simulink model "Kinematic_Delta_Robot"  (R2018b)
settings: Solver=VariableStepAuto  StartTime=0.0  StopTime=2  RelTol=1e-3
settings Model: Creator=User  LastModifiedBy=hugol
settings DebuggingCC: LibraryContextMissingDiagnostic=none
settings SFSimCC: SimUseLocalCustomCode=off
settings RTWCC: RTWUseLocalCustomCode=off
settings CodeAppCC: StateflowObjectComments=on

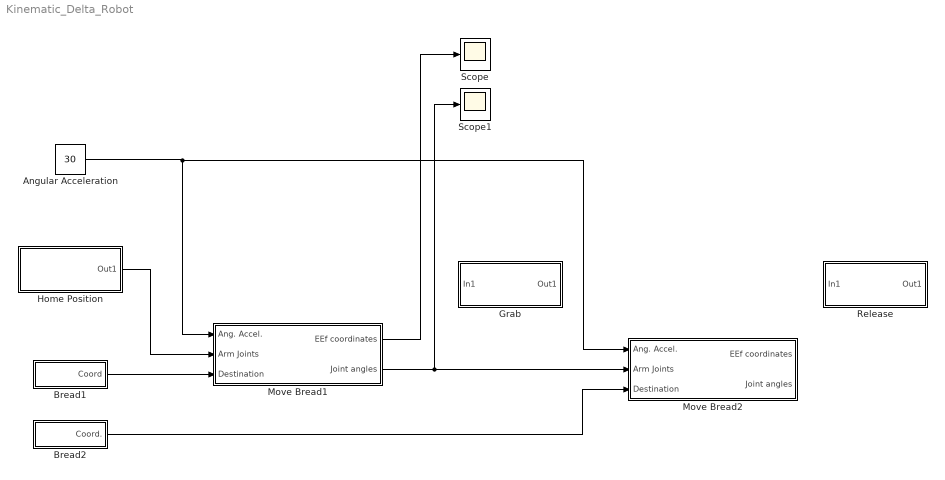
== system Kinematic_Delta_Robot ==
  Angular Acceleration : Constant  Value=30
  Bread1 : Subsystem
  Bread2 : Subsystem
  Grab : Subsystem
  Home Position : Subsystem
  Move Bread1 : Subsystem
  Move Bread2 : Subsystem
  Release : Subsystem
  Scope : Scope
  Scope1 : Scope
  wires:
  Bread1/1(Coord) -> Move Bread1/3(Destination)
  Home Position/1(Out1) -> Move Bread1/2(Arm Joints)
  Angular Acceleration/1 -> Move Bread2/1(Ang. Accel.), Move Bread1/1(Ang. Accel.)
  Bread2/1(Coord.) -> Move Bread2/3(Destination)
  Move Bread1/2(Joint angles) -> Scope1/1, Move Bread2/2(Arm Joints)
  Move Bread1/1(EEf coordinates) -> Scope/1

== system Kinematic_Delta_Robot/Bread1 ==
  Bread1.x : Constant  Value=48
  Bread1.y : Constant  Value=-25
  Bread1.z : Constant  Value=-400
  Mux : Mux  Inputs=3
  Coord : Outport
  wires:
  Bread1.y/1 -> Mux/2
  Bread1.z/1 -> Mux/3
  Bread1.x/1 -> Mux/1
  Mux/1 -> Coord/1

== system Kinematic_Delta_Robot/Bread2 ==
  Bread1.x : Constant  Value=48
  Bread1.y : Constant  Value=25
  Bread1.z : Constant  Value=-400
  Mux : Mux  Inputs=3
  Coord. : Outport
  wires:
  Bread1.y/1 -> Mux/2
  Bread1.z/1 -> Mux/3
  Bread1.x/1 -> Mux/1
  Mux/1 -> Coord./1

== system Kinematic_Delta_Robot/Grab ==
  In1 : Inport
  Out1 : Outport
  wires:
  In1/1 -> Out1/1

== system Kinematic_Delta_Robot/Home Position ==
  Arm1 : Constant  Value=0
  Arm2 : Constant  Value=-10
  Arm3 : Constant  Value=-5
  Mux : Mux  Inputs=3
  Out1 : Outport
  wires:
  Arm1/1 -> Mux/1
  Arm2/1 -> Mux/2
  Arm3/1 -> Mux/3
  Mux/1 -> Out1/1

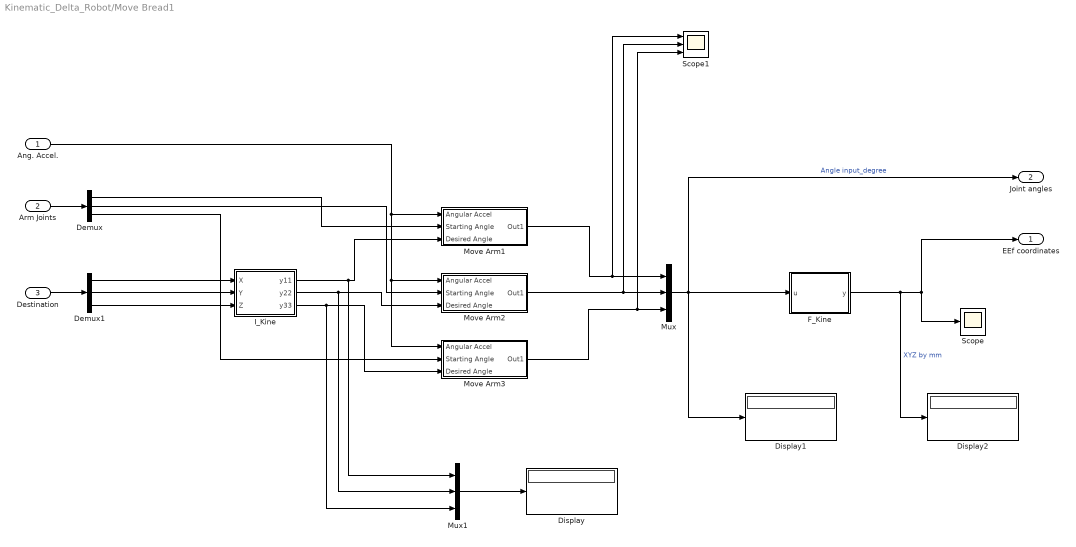
== system Kinematic_Delta_Robot/Move Bread1 ==
  Ang. Accel. : Inport
  Arm Joints : Inport  Port=2
  Destination : Inport  Port=3
  Demux : Demux  Outputs=3
  Demux1 : Demux  Outputs=3
  Display : Display
  Display1 : Display
  Display2 : Display
  F_Kine : MATLAB Function  TreatAsAtomicUnit=on
  I_Kine : MATLAB Function  TreatAsAtomicUnit=on
  Move Arm1 : Subsystem
  Move Arm2 : Subsystem
  Move Arm3 : Subsystem
  Mux : Mux  Inputs=3
  Mux1 : Mux  Inputs=3
  Scope : Scope
  Scope1 : Scope  NumInputPorts=3
  EEf coordinates : Outport
  Joint angles : Outport  Port=2
  wires:
  I_Kine/1(y11) -> Mux1/1, Move Arm1/3(Desired Angle)
  Demux/1 -> Move Arm1/2(Starting Angle)
  Move Arm3/1(Out1) -> Scope1/3, Mux/3
  Demux/2 -> Move Arm2/2(Starting Angle)
  Ang. Accel./1 -> Move Arm2/1(Angular Accel), Move Arm3/1(Angular Accel), Move Arm1/1(Angular Accel)
  Move Arm2/1(Out1) -> Scope1/2, Mux/2
  Move Arm1/1(Out1) -> Scope1/1, Mux/1
  Demux/3 -> Move Arm3/2(Starting Angle)
  I_Kine/2(y22) -> Move Arm2/3(Desired Angle), Mux1/2
  I_Kine/3(y33) -> Move Arm3/3(Desired Angle), Mux1/3
  Mux/1 -> Joint angles/1, Display1/1, F_Kine/1(u)  "Angle input_degree"
  F_Kine/1(y) -> Display2/1, EEf coordinates/1, Scope/1  "XYZ by mm"
  Mux1/1 -> Display/1
  Arm Joints/1 -> Demux/1
  Demux1/1 -> I_Kine/1(X)
  Demux1/2 -> I_Kine/2(Y)
  Demux1/3 -> I_Kine/3(Z)
  Destination/1 -> Demux1/1

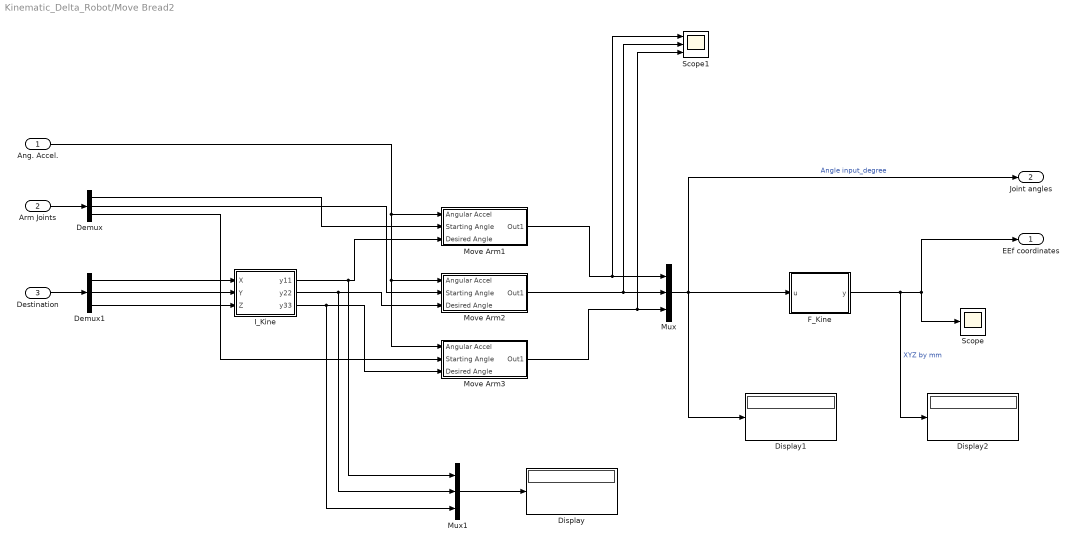
== system Kinematic_Delta_Robot/Move Bread2 ==
  Ang. Accel. : Inport
  Arm Joints : Inport  Port=2
  Destination : Inport  Port=3
  Demux : Demux  Outputs=3
  Demux1 : Demux  Outputs=3
  Display : Display
  Display1 : Display
  Display2 : Display
  F_Kine : MATLAB Function  TreatAsAtomicUnit=on
  I_Kine : MATLAB Function  TreatAsAtomicUnit=on
  Move Arm1 : Subsystem
  Move Arm2 : Subsystem
  Move Arm3 : Subsystem
  Mux : Mux  Inputs=3
  Mux1 : Mux  Inputs=3
  Scope : Scope
  Scope1 : Scope  NumInputPorts=3
  EEf coordinates : Outport
  Joint angles : Outport  Port=2
  wires:
  I_Kine/1(y11) -> Mux1/1, Move Arm1/3(Desired Angle)
  Demux/1 -> Move Arm1/2(Starting Angle)
  Move Arm3/1(Out1) -> Scope1/3, Mux/3
  Demux/2 -> Move Arm2/2(Starting Angle)
  Ang. Accel./1 -> Move Arm2/1(Angular Accel), Move Arm3/1(Angular Accel), Move Arm1/1(Angular Accel)
  Move Arm2/1(Out1) -> Scope1/2, Mux/2
  Move Arm1/1(Out1) -> Scope1/1, Mux/1
  Demux/3 -> Move Arm3/2(Starting Angle)
  I_Kine/2(y22) -> Move Arm2/3(Desired Angle), Mux1/2
  I_Kine/3(y33) -> Move Arm3/3(Desired Angle), Mux1/3
  Mux/1 -> Joint angles/1, Display1/1, F_Kine/1(u)  "Angle input_degree"
  F_Kine/1(y) -> Display2/1, EEf coordinates/1, Scope/1  "XYZ by mm"
  Mux1/1 -> Display/1
  Arm Joints/1 -> Demux/1
  Demux1/1 -> I_Kine/1(X)
  Demux1/2 -> I_Kine/2(Y)
  Demux1/3 -> I_Kine/3(Z)
  Destination/1 -> Demux1/1

== system Kinematic_Delta_Robot/Release ==
  In1 : Inport
  Out1 : Outport
  wires:
  In1/1 -> Out1/1

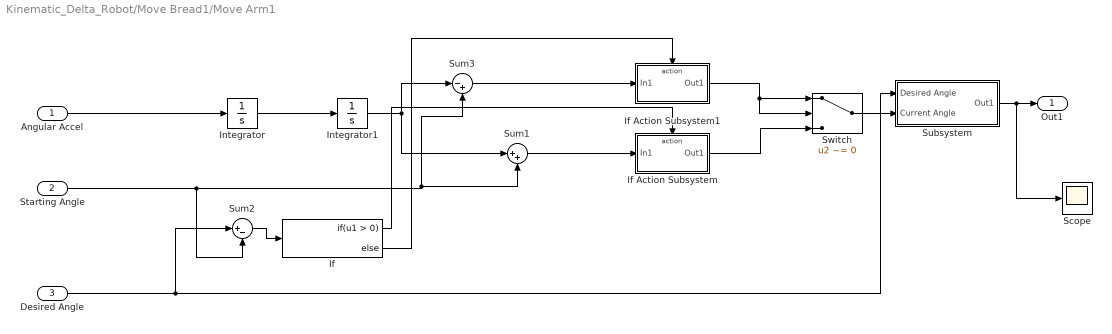
== system Kinematic_Delta_Robot/Move Bread1/Move Arm1 ==
  Angular Accel : Inport
  Starting Angle : Inport  Port=2
  Desired Angle : Inport  Port=3
  If : If
  If Action Subsystem : Subsystem  TreatAsAtomicUnit=on
  If Action Subsystem1 : Subsystem  TreatAsAtomicUnit=on
  Integrator : Integrator
  Integrator1 : Integrator
  Scope : Scope
  Subsystem : Subsystem
  Sum1 : Sum  Inputs=|++
  Sum2 : Sum  Inputs=|+-
  Sum3 : Sum  Inputs=|-+
  Switch : Switch  Criteria=u2 ~= 0
  Out1 : Outport
  wires:
  Angular Accel/1 -> Integrator/1
  Integrator/1 -> Integrator1/1
  If Action Subsystem/1(Out1) -> Switch/3
  Sum2/1 -> If/1
  If/2 -> If Action Subsystem1/Action
  Starting Angle/1 -> Sum2/2, Sum3/2, Sum1/2
  Desired Angle/1 -> Subsystem/1(Desired Angle), Sum2/1
  If Action Subsystem1/1(Out1) -> Switch/1, Switch/2
  If/1 -> If Action Subsystem/Action
  Integrator1/1 -> Sum1/1, Sum3/1
  Sum3/1 -> If Action Subsystem1/1(In1)
  Sum1/1 -> If Action Subsystem/1(In1)
  Switch/1 -> Subsystem/2(Current Angle)
  Subsystem/1(Out1) -> Scope/1, Out1/1

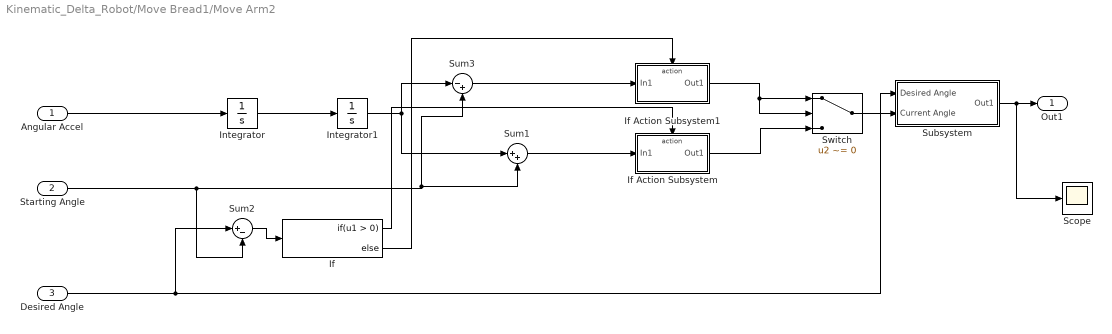
== system Kinematic_Delta_Robot/Move Bread1/Move Arm2 ==
  Angular Accel : Inport
  Starting Angle : Inport  Port=2
  Desired Angle : Inport  Port=3
  If : If
  If Action Subsystem : Subsystem  TreatAsAtomicUnit=on
  If Action Subsystem1 : Subsystem  TreatAsAtomicUnit=on
  Integrator : Integrator
  Integrator1 : Integrator
  Scope : Scope
  Subsystem : Subsystem
  Sum1 : Sum  Inputs=|++
  Sum2 : Sum  Inputs=|+-
  Sum3 : Sum  Inputs=|-+
  Switch : Switch  Criteria=u2 ~= 0
  Out1 : Outport
  wires:
  Angular Accel/1 -> Integrator/1
  Integrator/1 -> Integrator1/1
  If Action Subsystem/1(Out1) -> Switch/3
  Sum2/1 -> If/1
  If/2 -> If Action Subsystem1/Action
  Starting Angle/1 -> Sum2/2, Sum3/2, Sum1/2
  Desired Angle/1 -> Subsystem/1(Desired Angle), Sum2/1
  If Action Subsystem1/1(Out1) -> Switch/1, Switch/2
  If/1 -> If Action Subsystem/Action
  Integrator1/1 -> Sum1/1, Sum3/1
  Sum3/1 -> If Action Subsystem1/1(In1)
  Sum1/1 -> If Action Subsystem/1(In1)
  Switch/1 -> Subsystem/2(Current Angle)
  Subsystem/1(Out1) -> Scope/1, Out1/1

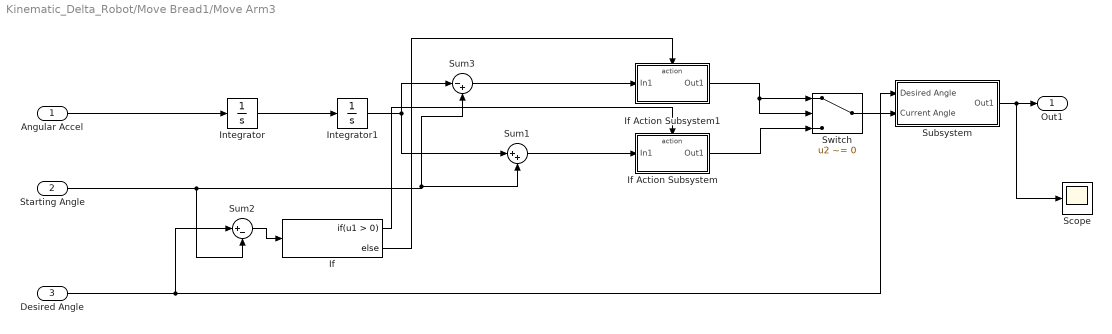
== system Kinematic_Delta_Robot/Move Bread1/Move Arm3 ==
  Angular Accel : Inport
  Starting Angle : Inport  Port=2
  Desired Angle : Inport  Port=3
  If : If
  If Action Subsystem : Subsystem  TreatAsAtomicUnit=on
  If Action Subsystem1 : Subsystem  TreatAsAtomicUnit=on
  Integrator : Integrator
  Integrator1 : Integrator
  Scope : Scope
  Subsystem : Subsystem
  Sum1 : Sum  Inputs=|++
  Sum2 : Sum  Inputs=|+-
  Sum3 : Sum  Inputs=|-+
  Switch : Switch  Criteria=u2 ~= 0
  Out1 : Outport
  wires:
  Angular Accel/1 -> Integrator/1
  Integrator/1 -> Integrator1/1
  If Action Subsystem/1(Out1) -> Switch/3
  Sum2/1 -> If/1
  If/2 -> If Action Subsystem1/Action
  Starting Angle/1 -> Sum2/2, Sum3/2, Sum1/2
  Desired Angle/1 -> Subsystem/1(Desired Angle), Sum2/1
  If Action Subsystem1/1(Out1) -> Switch/1, Switch/2
  If/1 -> If Action Subsystem/Action
  Integrator1/1 -> Sum1/1, Sum3/1
  Sum3/1 -> If Action Subsystem1/1(In1)
  Sum1/1 -> If Action Subsystem/1(In1)
  Switch/1 -> Subsystem/2(Current Angle)
  Subsystem/1(Out1) -> Scope/1, Out1/1

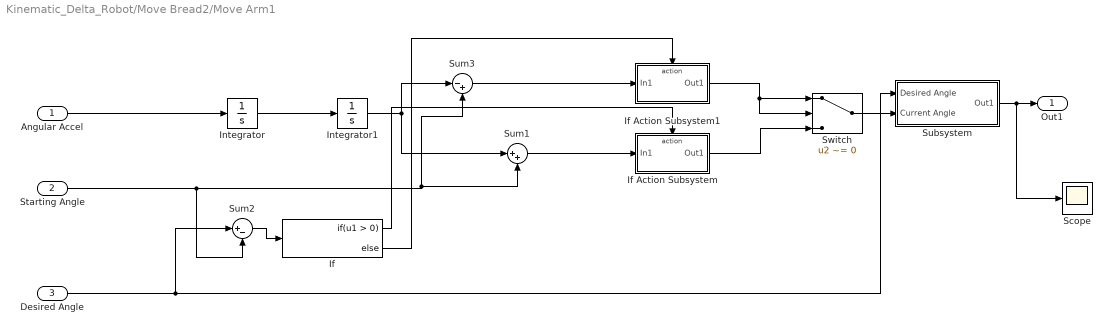
== system Kinematic_Delta_Robot/Move Bread2/Move Arm1 ==
  Angular Accel : Inport
  Starting Angle : Inport  Port=2
  Desired Angle : Inport  Port=3
  If : If
  If Action Subsystem : Subsystem  TreatAsAtomicUnit=on
  If Action Subsystem1 : Subsystem  TreatAsAtomicUnit=on
  Integrator : Integrator
  Integrator1 : Integrator
  Scope : Scope
  Subsystem : Subsystem
  Sum1 : Sum  Inputs=|++
  Sum2 : Sum  Inputs=|+-
  Sum3 : Sum  Inputs=|-+
  Switch : Switch  Criteria=u2 ~= 0
  Out1 : Outport
  wires:
  Angular Accel/1 -> Integrator/1
  Integrator/1 -> Integrator1/1
  If Action Subsystem/1(Out1) -> Switch/3
  Sum2/1 -> If/1
  If/2 -> If Action Subsystem1/Action
  Starting Angle/1 -> Sum2/2, Sum3/2, Sum1/2
  Desired Angle/1 -> Subsystem/1(Desired Angle), Sum2/1
  If Action Subsystem1/1(Out1) -> Switch/1, Switch/2
  If/1 -> If Action Subsystem/Action
  Integrator1/1 -> Sum1/1, Sum3/1
  Sum3/1 -> If Action Subsystem1/1(In1)
  Sum1/1 -> If Action Subsystem/1(In1)
  Switch/1 -> Subsystem/2(Current Angle)
  Subsystem/1(Out1) -> Scope/1, Out1/1

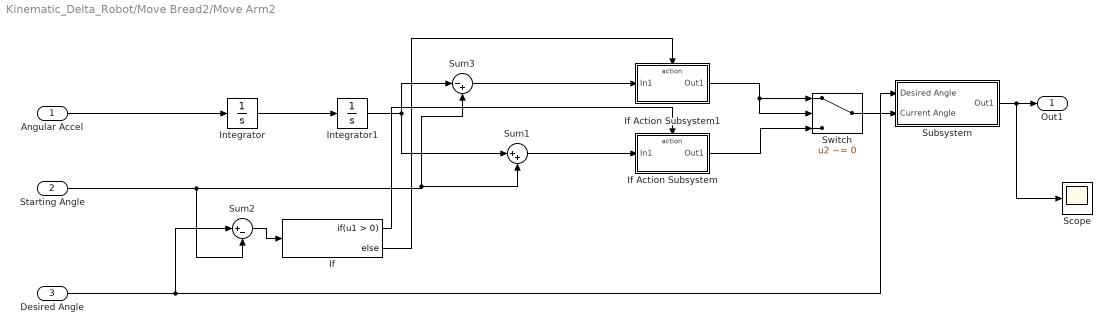
== system Kinematic_Delta_Robot/Move Bread2/Move Arm2 ==
  Angular Accel : Inport
  Starting Angle : Inport  Port=2
  Desired Angle : Inport  Port=3
  If : If
  If Action Subsystem : Subsystem  TreatAsAtomicUnit=on
  If Action Subsystem1 : Subsystem  TreatAsAtomicUnit=on
  Integrator : Integrator
  Integrator1 : Integrator
  Scope : Scope
  Subsystem : Subsystem
  Sum1 : Sum  Inputs=|++
  Sum2 : Sum  Inputs=|+-
  Sum3 : Sum  Inputs=|-+
  Switch : Switch  Criteria=u2 ~= 0
  Out1 : Outport
  wires:
  Angular Accel/1 -> Integrator/1
  Integrator/1 -> Integrator1/1
  If Action Subsystem/1(Out1) -> Switch/3
  Sum2/1 -> If/1
  If/2 -> If Action Subsystem1/Action
  Starting Angle/1 -> Sum2/2, Sum3/2, Sum1/2
  Desired Angle/1 -> Subsystem/1(Desired Angle), Sum2/1
  If Action Subsystem1/1(Out1) -> Switch/1, Switch/2
  If/1 -> If Action Subsystem/Action
  Integrator1/1 -> Sum1/1, Sum3/1
  Sum3/1 -> If Action Subsystem1/1(In1)
  Sum1/1 -> If Action Subsystem/1(In1)
  Switch/1 -> Subsystem/2(Current Angle)
  Subsystem/1(Out1) -> Scope/1, Out1/1

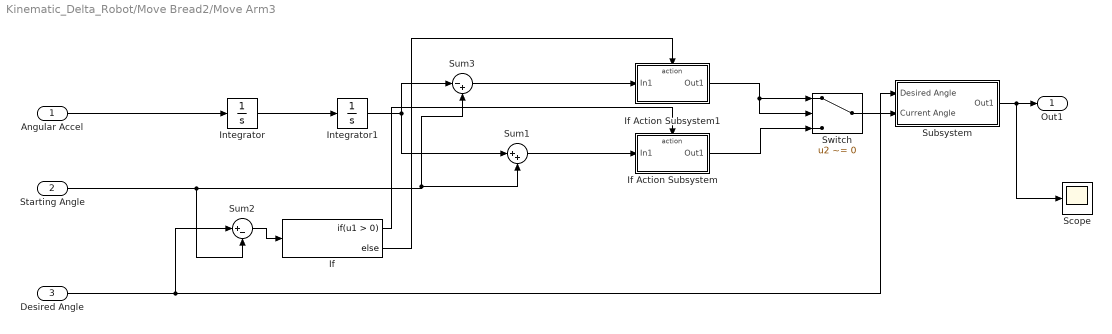
== system Kinematic_Delta_Robot/Move Bread2/Move Arm3 ==
  Angular Accel : Inport
  Starting Angle : Inport  Port=2
  Desired Angle : Inport  Port=3
  If : If
  If Action Subsystem : Subsystem  TreatAsAtomicUnit=on
  If Action Subsystem1 : Subsystem  TreatAsAtomicUnit=on
  Integrator : Integrator
  Integrator1 : Integrator
  Scope : Scope
  Subsystem : Subsystem
  Sum1 : Sum  Inputs=|++
  Sum2 : Sum  Inputs=|+-
  Sum3 : Sum  Inputs=|-+
  Switch : Switch  Criteria=u2 ~= 0
  Out1 : Outport
  wires:
  Angular Accel/1 -> Integrator/1
  Integrator/1 -> Integrator1/1
  If Action Subsystem/1(Out1) -> Switch/3
  Sum2/1 -> If/1
  If/2 -> If Action Subsystem1/Action
  Starting Angle/1 -> Sum2/2, Sum3/2, Sum1/2
  Desired Angle/1 -> Subsystem/1(Desired Angle), Sum2/1
  If Action Subsystem1/1(Out1) -> Switch/1, Switch/2
  If/1 -> If Action Subsystem/Action
  Integrator1/1 -> Sum1/1, Sum3/1
  Sum3/1 -> If Action Subsystem1/1(In1)
  Sum1/1 -> If Action Subsystem/1(In1)
  Switch/1 -> Subsystem/2(Current Angle)
  Subsystem/1(Out1) -> Scope/1, Out1/1

== system Kinematic_Delta_Robot/Move Bread1/Move Arm1/If Action Subsystem ==
  In1 : Inport
  Action Port : ActionPort  ActionType=then
  Out1 : Outport
  wires:
  In1/1 -> Out1/1

== system Kinematic_Delta_Robot/Move Bread1/Move Arm1/If Action Subsystem1 ==
  In1 : Inport
  Action Port : ActionPort  ActionType=else
  Out1 : Outport
  wires:
  In1/1 -> Out1/1

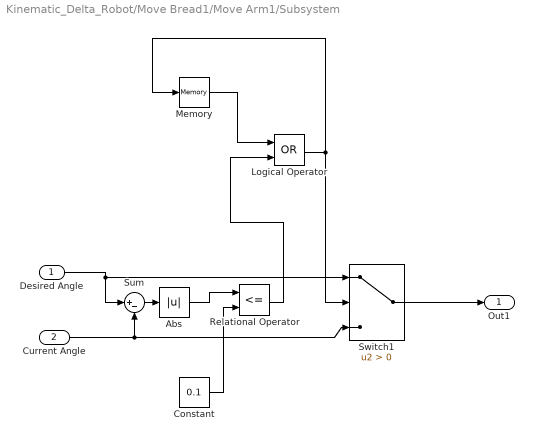
== system Kinematic_Delta_Robot/Move Bread1/Move Arm1/Subsystem ==
  Desired Angle : Inport
  Current Angle : Inport  Port=2
  Abs : Abs
  Constant : Constant  Value=0.1
  Logical Operator : Logic  Operator=OR  AllPortsSameDT=off  OutDataTypeStr=boolean
  Memory : Memory
  Relational Operator : RelationalOperator  Operator=<=  OutDataTypeStr=boolean  RndMeth=Simplest
  Sum : Sum  Inputs=|+-
  Switch1 : Switch  Criteria=u2 > Threshold
  Out1 : Outport
  wires:
  Switch1/1 -> Out1/1
  Desired Angle/1 -> Sum/1, Switch1/1
  Current Angle/1 -> Switch1/3, Sum/2
  Sum/1 -> Abs/1
  Abs/1 -> Relational Operator/1
  Constant/1 -> Relational Operator/2
  Relational Operator/1 -> Logical Operator/2
  Logical Operator/1 -> Memory/1, Switch1/2
  Memory/1 -> Logical Operator/1

== system Kinematic_Delta_Robot/Move Bread1/Move Arm2/If Action Subsystem ==
  In1 : Inport
  Action Port : ActionPort  ActionType=then
  Out1 : Outport
  wires:
  In1/1 -> Out1/1

== system Kinematic_Delta_Robot/Move Bread1/Move Arm2/If Action Subsystem1 ==
  In1 : Inport
  Action Port : ActionPort  ActionType=else
  Out1 : Outport
  wires:
  In1/1 -> Out1/1

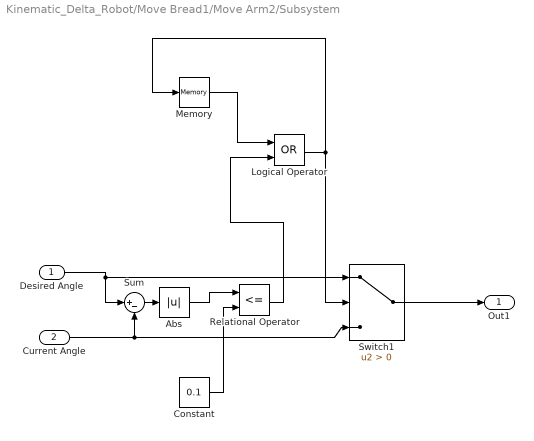
== system Kinematic_Delta_Robot/Move Bread1/Move Arm2/Subsystem ==
  Desired Angle : Inport
  Current Angle : Inport  Port=2
  Abs : Abs
  Constant : Constant  Value=0.1
  Logical Operator : Logic  Operator=OR  AllPortsSameDT=off  OutDataTypeStr=boolean
  Memory : Memory
  Relational Operator : RelationalOperator  Operator=<=  OutDataTypeStr=boolean  RndMeth=Simplest
  Sum : Sum  Inputs=|+-
  Switch1 : Switch  Criteria=u2 > Threshold
  Out1 : Outport
  wires:
  Switch1/1 -> Out1/1
  Desired Angle/1 -> Sum/1, Switch1/1
  Current Angle/1 -> Switch1/3, Sum/2
  Sum/1 -> Abs/1
  Abs/1 -> Relational Operator/1
  Constant/1 -> Relational Operator/2
  Relational Operator/1 -> Logical Operator/2
  Logical Operator/1 -> Memory/1, Switch1/2
  Memory/1 -> Logical Operator/1

== system Kinematic_Delta_Robot/Move Bread1/Move Arm3/If Action Subsystem ==
  In1 : Inport
  Action Port : ActionPort  ActionType=then
  Out1 : Outport
  wires:
  In1/1 -> Out1/1

== system Kinematic_Delta_Robot/Move Bread1/Move Arm3/If Action Subsystem1 ==
  In1 : Inport
  Action Port : ActionPort  ActionType=else
  Out1 : Outport
  wires:
  In1/1 -> Out1/1

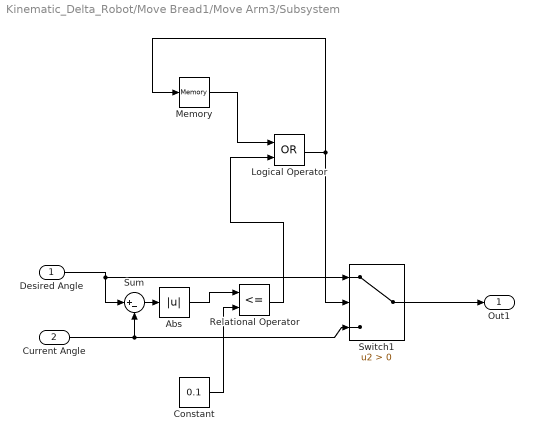
== system Kinematic_Delta_Robot/Move Bread1/Move Arm3/Subsystem ==
  Desired Angle : Inport
  Current Angle : Inport  Port=2
  Abs : Abs
  Constant : Constant  Value=0.1
  Logical Operator : Logic  Operator=OR  AllPortsSameDT=off  OutDataTypeStr=boolean
  Memory : Memory
  Relational Operator : RelationalOperator  Operator=<=  OutDataTypeStr=boolean  RndMeth=Simplest
  Sum : Sum  Inputs=|+-
  Switch1 : Switch  Criteria=u2 > Threshold
  Out1 : Outport
  wires:
  Switch1/1 -> Out1/1
  Desired Angle/1 -> Sum/1, Switch1/1
  Current Angle/1 -> Switch1/3, Sum/2
  Sum/1 -> Abs/1
  Abs/1 -> Relational Operator/1
  Constant/1 -> Relational Operator/2
  Relational Operator/1 -> Logical Operator/2
  Logical Operator/1 -> Memory/1, Switch1/2
  Memory/1 -> Logical Operator/1

== system Kinematic_Delta_Robot/Move Bread2/Move Arm1/If Action Subsystem ==
  In1 : Inport
  Action Port : ActionPort  ActionType=then
  Out1 : Outport
  wires:
  In1/1 -> Out1/1

== system Kinematic_Delta_Robot/Move Bread2/Move Arm1/If Action Subsystem1 ==
  In1 : Inport
  Action Port : ActionPort  ActionType=else
  Out1 : Outport
  wires:
  In1/1 -> Out1/1

== system Kinematic_Delta_Robot/Move Bread2/Move Arm1/Subsystem ==
  Desired Angle : Inport
  Current Angle : Inport  Port=2
  Abs : Abs
  Constant : Constant  Value=0.1
  Logical Operator : Logic  Operator=OR  AllPortsSameDT=off  OutDataTypeStr=boolean
  Memory : Memory
  Relational Operator : RelationalOperator  Operator=<=  OutDataTypeStr=boolean  RndMeth=Simplest
  Sum : Sum  Inputs=|+-
  Switch1 : Switch  Criteria=u2 > Threshold
  Out1 : Outport
  wires:
  Switch1/1 -> Out1/1
  Desired Angle/1 -> Sum/1, Switch1/1
  Current Angle/1 -> Switch1/3, Sum/2
  Sum/1 -> Abs/1
  Abs/1 -> Relational Operator/1
  Constant/1 -> Relational Operator/2
  Relational Operator/1 -> Logical Operator/2
  Logical Operator/1 -> Memory/1, Switch1/2
  Memory/1 -> Logical Operator/1

== system Kinematic_Delta_Robot/Move Bread2/Move Arm2/If Action Subsystem ==
  In1 : Inport
  Action Port : ActionPort  ActionType=then
  Out1 : Outport
  wires:
  In1/1 -> Out1/1

== system Kinematic_Delta_Robot/Move Bread2/Move Arm2/If Action Subsystem1 ==
  In1 : Inport
  Action Port : ActionPort  ActionType=else
  Out1 : Outport
  wires:
  In1/1 -> Out1/1

== system Kinematic_Delta_Robot/Move Bread2/Move Arm2/Subsystem ==
  Desired Angle : Inport
  Current Angle : Inport  Port=2
  Abs : Abs
  Constant : Constant  Value=0.1
  Logical Operator : Logic  Operator=OR  AllPortsSameDT=off  OutDataTypeStr=boolean
  Memory : Memory
  Relational Operator : RelationalOperator  Operator=<=  OutDataTypeStr=boolean  RndMeth=Simplest
  Sum : Sum  Inputs=|+-
  Switch1 : Switch  Criteria=u2 > Threshold
  Out1 : Outport
  wires:
  Switch1/1 -> Out1/1
  Desired Angle/1 -> Sum/1, Switch1/1
  Current Angle/1 -> Switch1/3, Sum/2
  Sum/1 -> Abs/1
  Abs/1 -> Relational Operator/1
  Constant/1 -> Relational Operator/2
  Relational Operator/1 -> Logical Operator/2
  Logical Operator/1 -> Memory/1, Switch1/2
  Memory/1 -> Logical Operator/1

== system Kinematic_Delta_Robot/Move Bread2/Move Arm3/If Action Subsystem ==
  In1 : Inport
  Action Port : ActionPort  ActionType=then
  Out1 : Outport
  wires:
  In1/1 -> Out1/1

== system Kinematic_Delta_Robot/Move Bread2/Move Arm3/If Action Subsystem1 ==
  In1 : Inport
  Action Port : ActionPort  ActionType=else
  Out1 : Outport
  wires:
  In1/1 -> Out1/1

== system Kinematic_Delta_Robot/Move Bread2/Move Arm3/Subsystem ==
  Desired Angle : Inport
  Current Angle : Inport  Port=2
  Abs : Abs
  Constant : Constant  Value=0.1
  Logical Operator : Logic  Operator=OR  AllPortsSameDT=off  OutDataTypeStr=boolean
  Memory : Memory
  Relational Operator : RelationalOperator  Operator=<=  OutDataTypeStr=boolean  RndMeth=Simplest
  Sum : Sum  Inputs=|+-
  Switch1 : Switch  Criteria=u2 > Threshold
  Out1 : Outport
  wires:
  Switch1/1 -> Out1/1
  Desired Angle/1 -> Sum/1, Switch1/1
  Current Angle/1 -> Switch1/3, Sum/2
  Sum/1 -> Abs/1
  Abs/1 -> Relational Operator/1
  Constant/1 -> Relational Operator/2
  Relational Operator/1 -> Logical Operator/2
  Logical Operator/1 -> Memory/1, Switch1/2
  Memory/1 -> Logical Operator/1

== matlab function Kinematic_Delta_Robot/Move Bread1/I_Kine ==
  data: X input; y11 output; Y input; Z input; y22 output; y33 output
% By Hasan Zabihifar in Skoltech_2017

function [y11,y22,y33] = fcn(X,Y,Z)
u1=X;
u2=Y;
u3=Z;

f  =  38;
rf =  127;
re = 400;
e  =  38;




sqrt3 = sqrt(3.0);
pi     = 3.141592653;
sin120 = sqrt3 / 2.0;
cos120 = -0.5;
tan60  = sqrt3;
sin30  = 0.5;
tan30  = 1.0 / sqrt3;

%..................................................... Inverse Kinematics
    x0 =u1;
    y0 =u2;
    z0 =u3;

    y1 = -0.5*0.57735*f ;
    y0 = y0-0.5*0.57735*e; % shift center to edge
    
    a = (x0.*x0 + y0.*y0 + z0.*z0 + rf.*rf - re.*re - y1.*y1) ./ (2.0.*z0);
    b = (y1-y0) ./ z0;

    % discriminant
    d = -(a + b.*y1).*(a + b.*y1) + rf.*(b.*b.*rf + rf);
   
   
    yj = (y1 - a.*b - sqrt(d)) ./ (b.*b + 1); 
    zj = a + b.*yj;
    if yj>y1 
        p=180;
    else
        p=0;
    end
    theta = atan(-zj ./ (y1-yj)) .* 180.0 / pi + p;
     
    y11=theta;
    
    if d<0 
        y11=0; % non-existing povar. 
        
    end  
    %.......................................................
    x0 =u1*cos120 + u2*sin120;
    y0 =u2*cos120-u1*sin120;
    z0 =u3;

    y1 = -0.5*0.57735*f ;
    y0 = y0-0.5*0.57735*e; % shift center to edge
    % z = a + b*y
    a = (x0.*x0 + y0.*y0 + z0.*z0 + rf.*rf - re.*re - y1.*y1) ./ (2.0.*z0);
    b = (y1-y0) ./ z0;

    % discriminant
    d = -(a + b.*y1).*(a + b.*y1) + rf.*(b.*b.*rf + rf);
  
    yj = (y1 - a.*b - sqrt(d)) ./ (b.*b + 1); % choosing outer povar
    zj = a + b.*yj;
    if yj>y1 
        p=180;
    else
        p=0;
    end
    theta = atan(-zj ./ (y1-yj)) .* 180.0 / pi + p;
    y22=theta;
   
    if d<0 
        y22=0; % non-existing povar.
        
    end 
    %.......................................................
     x0 =u1*cos120 - u2*sin120;
    y0 =u2*cos120+u1*sin120;
    z0 =u3;

    y1 = -0.5*0.57735*f ;
    y0 = y0-0.5*0.57735*e; % shift center to edge
    % z = a + b*y
    a = (x0.*x0 + y0.*y0 + z0.*z0 + rf.*rf - re.*re - y1.*y1) ./ (2.0.*z0);
    b = (y1-y0) ./ z0;

    % discriminant
    d = -(a + b.*y1).*(a + b.*y1) + rf.*(b.*b.*rf + rf);
  
    yj = (y1 - a.*b - sqrt(d)) ./ (b.*b + 1); % choosing outer povar
    zj = a + b.*yj;
    if yj>y1 
        p=180;
    else
        p=0;
    end
    theta = atan(-zj ./ (y1-yj)) .* 180.0 / pi + p;
    
   y33=theta; % return error, theta
     if d<0 
        y33=0; % non-existing povar.  
        
    end 
end

== matlab function Kinematic_Delta_Robot/Move Bread1/F_Kine ==
  data: u input; y output
% By Hasan Zabihifar in Skoltech_2017

function y = fcn(u)

f  =  38;
rf =  127;
re = 400;
e  =  38;

sqrt3 = sqrt(3.0);
pi     = 3.141592653;
sin120 = sqrt3 / 2.0;
cos120 = -0.5;
tan60  = sqrt3;
sin30  = 0.5;
tan30  = 1.0 / sqrt3;

%..................................................... Forward Kinematics
    theta1 =u(1);
    theta2 =u(2);
    theta3 =u(3);
    
    t = (f-e) * tan30 / 2.0;
    dtr = pi / 180.0;
    
    theta1 =theta1.*dtr;
    theta2 =theta2.*dtr;
    theta3 =theta3.*dtr;
    
    y1 = -(t + rf.*cos(theta1) );
    z1 = -rf .* sin(theta1);
    
    y2 = (t + rf.*cos(theta2)) .* sin30;
    x2 = y2 .* tan60;
    z2 = -rf .* sin(theta2);
    
    y3 = (t + rf.*cos(theta3)) .* sin30;
    x3 = -y3 .* tan60;
    z3 = -rf .* sin(theta3);
    
    dnm = (y2-y1).*x3 - (y3-y1).*x2;
    
    w1 = y1.*y1 + z1.*z1;
    w2 = x2.*x2 + y2.*y2 + z2.*z2;
    w3 = x3.*x3 + y3.*y3 + z3.*z3;
    
    % x = (a1*z + b1)/dnm
    a1 = (z2-z1).*(y3-y1) - (z3-z1).*(y2-y1);
    b1= -( (w2-w1).*(y3-y1) - (w3-w1).*(y2-y1) ) ./ 2.0;
    
    % y = (a2*z + b2)/dnm
    a2 = -(z2-z1).*x3 + (z3-z1).*x2;
    b2 = ( (w2-w1).*x3 - (w3-w1).*x2) ./ 2.0;
    
    % a*z^2 + b*z + c = 0
    a = a1.*a1 + a2.*a2 + dnm.*dnm;
    b = 2.0 .* (a1.*b1 + a2.*(b2 - y1.*dnm) - z1.*dnm.*dnm);
    c = (b2 - y1.*dnm).*(b2 - y1.*dnm) + b1.*b1 + dnm.*dnm.*(z1.*z1 - re.*re);
    
    % discriminant
    d = b.*b - 4.0.*a.*c;
    if d < 0.0
        y= [0,0,0]; % non-existing povar. 
    
    else
    z0 = -0.5.*(b + sqrt(d)) ./ a;
    x0 = (a1.*z0 + b1) ./ dnm;
    y0 = (a2.*z0 + b2) ./ dnm;

    y =[x0,y0,z0];
    end
    end

== matlab function Kinematic_Delta_Robot/Move Bread2/F_Kine ==
  data: u input; y output
% By Hasan Zabihifar in Skoltech_2017

function y = fcn(u)

f  =  38;
rf =  127;
re = 400;
e  =  38;

sqrt3 = sqrt(3.0);
pi     = 3.141592653;
sin120 = sqrt3 / 2.0;
cos120 = -0.5;
tan60  = sqrt3;
sin30  = 0.5;
tan30  = 1.0 / sqrt3;

%..................................................... Forward Kinematics
    theta1 =u(1);
    theta2 =u(2);
    theta3 =u(3);
    
    t = (f-e) * tan30 / 2.0;
    dtr = pi / 180.0;
    
    theta1 =theta1.*dtr;
    theta2 =theta2.*dtr;
    theta3 =theta3.*dtr;
    
    y1 = -(t + rf.*cos(theta1) );
    z1 = -rf .* sin(theta1);
    
    y2 = (t + rf.*cos(theta2)) .* sin30;
    x2 = y2 .* tan60;
    z2 = -rf .* sin(theta2);
    
    y3 = (t + rf.*cos(theta3)) .* sin30;
    x3 = -y3 .* tan60;
    z3 = -rf .* sin(theta3);
    
    dnm = (y2-y1).*x3 - (y3-y1).*x2;
    
    w1 = y1.*y1 + z1.*z1;
    w2 = x2.*x2 + y2.*y2 + z2.*z2;
    w3 = x3.*x3 + y3.*y3 + z3.*z3;
    
    % x = (a1*z + b1)/dnm
    a1 = (z2-z1).*(y3-y1) - (z3-z1).*(y2-y1);
    b1= -( (w2-w1).*(y3-y1) - (w3-w1).*(y2-y1) ) ./ 2.0;
    
    % y = (a2*z + b2)/dnm
    a2 = -(z2-z1).*x3 + (z3-z1).*x2;
    b2 = ( (w2-w1).*x3 - (w3-w1).*x2) ./ 2.0;
    
    % a*z^2 + b*z + c = 0
    a = a1.*a1 + a2.*a2 + dnm.*dnm;
    b = 2.0 .* (a1.*b1 + a2.*(b2 - y1.*dnm) - z1.*dnm.*dnm);
    c = (b2 - y1.*dnm).*(b2 - y1.*dnm) + b1.*b1 + dnm.*dnm.*(z1.*z1 - re.*re);
    
    % discriminant
    d = b.*b - 4.0.*a.*c;
    if d < 0.0
        y= [0,0,0]; % non-existing povar. 
    
    else
    z0 = -0.5.*(b + sqrt(d)) ./ a;
    x0 = (a1.*z0 + b1) ./ dnm;
    y0 = (a2.*z0 + b2) ./ dnm;

    y =[x0,y0,z0];
    end
    end

== matlab function Kinematic_Delta_Robot/Move Bread2/I_Kine ==
  data: X input; y11 output; Y input; Z input; y22 output; y33 output
% By Hasan Zabihifar in Skoltech_2017

function [y11,y22,y33] = fcn(X,Y,Z)
u1=X;
u2=Y;
u3=Z;

f  =  38;
rf =  127;
re = 400;
e  =  38;




sqrt3 = sqrt(3.0);
pi     = 3.141592653;
sin120 = sqrt3 / 2.0;
cos120 = -0.5;
tan60  = sqrt3;
sin30  = 0.5;
tan30  = 1.0 / sqrt3;

%..................................................... Inverse Kinematics
    x0 =u1;
    y0 =u2;
    z0 =u3;

    y1 = -0.5*0.57735*f ;
    y0 = y0-0.5*0.57735*e; % shift center to edge
    
    a = (x0.*x0 + y0.*y0 + z0.*z0 + rf.*rf - re.*re - y1.*y1) ./ (2.0.*z0);
    b = (y1-y0) ./ z0;

    % discriminant
    d = -(a + b.*y1).*(a + b.*y1) + rf.*(b.*b.*rf + rf);
   
   
    yj = (y1 - a.*b - sqrt(d)) ./ (b.*b + 1); 
    zj = a + b.*yj;
    if yj>y1 
        p=180;
    else
        p=0;
    end
    theta = atan(-zj ./ (y1-yj)) .* 180.0 / pi + p;
     
    y11=theta;
    
    if d<0 
        y11=0; % non-existing povar. 
        
    end  
    %.......................................................
    x0 =u1*cos120 + u2*sin120;
    y0 =u2*cos120-u1*sin120;
    z0 =u3;

    y1 = -0.5*0.57735*f ;
    y0 = y0-0.5*0.57735*e; % shift center to edge
    % z = a + b*y
    a = (x0.*x0 + y0.*y0 + z0.*z0 + rf.*rf - re.*re - y1.*y1) ./ (2.0.*z0);
    b = (y1-y0) ./ z0;

    % discriminant
    d = -(a + b.*y1).*(a + b.*y1) + rf.*(b.*b.*rf + rf);
  
    yj = (y1 - a.*b - sqrt(d)) ./ (b.*b + 1); % choosing outer povar
    zj = a + b.*yj;
    if yj>y1 
        p=180;
    else
        p=0;
    end
    theta = atan(-zj ./ (y1-yj)) .* 180.0 / pi + p;
    y22=theta;
   
    if d<0 
        y22=0; % non-existing povar.
        
    end 
    %.......................................................
     x0 =u1*cos120 - u2*sin120;
    y0 =u2*cos120+u1*sin120;
    z0 =u3;

    y1 = -0.5*0.57735*f ;
    y0 = y0-0.5*0.57735*e; % shift center to edge
    % z = a + b*y
    a = (x0.*x0 + y0.*y0 + z0.*z0 + rf.*rf - re.*re - y1.*y1) ./ (2.0.*z0);
    b = (y1-y0) ./ z0;

    % discriminant
    d = -(a + b.*y1).*(a + b.*y1) + rf.*(b.*b.*rf + rf);
  
    yj = (y1 - a.*b - sqrt(d)) ./ (b.*b + 1); % choosing outer povar
    zj = a + b.*yj;
    if yj>y1 
        p=180;
    else
        p=0;
    end
    theta = atan(-zj ./ (y1-yj)) .* 180.0 / pi + p;
    
   y33=theta; % return error, theta
     if d<0 
        y33=0; % non-existing povar.  
        
    end 
end
